simulink model "step1"  (R2021a)
settings: Solver=FixedStepAuto  StartTime=0.0  StopTime=100.0  FixedStep=0.001  RelTol=1e-3
settings Model: Creator=konsta  LastModifiedBy=konsta

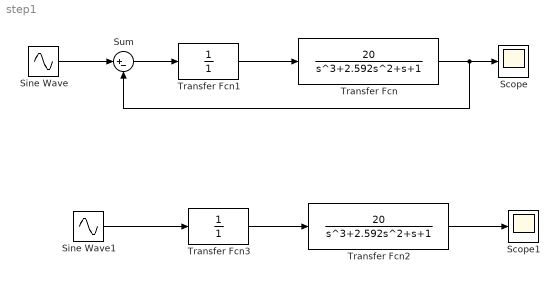
== system step1 ==
  Scope : Scope
  Scope1 : Scope
  Sine Wave : Sin  SampleTime=0
  Sine Wave1 : Sin  SampleTime=0
  Sum : Sum  Inputs=|+-
  Transfer Fcn : TransferFcn  Numerator=[20]  Denominator=[1 2.592 1 1]
  Transfer Fcn1 : TransferFcn  Denominator=[0 1]
  Transfer Fcn2 : TransferFcn  Numerator=[20]  Denominator=[1 2.592 1 1]
  Transfer Fcn3 : TransferFcn  Denominator=[0 1]
  wires:
  Sine Wave/1 -> Sum/1
  Sum/1 -> Transfer Fcn1/1
  Transfer Fcn1/1 -> Transfer Fcn/1
  Transfer Fcn/1 -> Sum/2, Scope/1
  Transfer Fcn3/1 -> Transfer Fcn2/1
  Transfer Fcn2/1 -> Scope1/1
  Sine Wave1/1 -> Transfer Fcn3/1
